simulink model "SimulacionControladorRechazoPerturbacion"  (R2023b)
settings: Solver=VariableStepAuto  StartTime=0.0  StopTime=30  RelTol=1e-3
values from neighbouring files (symbols this model uses):
  alfa_cu = 3.9E-3    (= 0.0039)    [Parametros.m]
  b_a = J_eq * n * omega_n    [MigracionPolosControladorExterno.m]    (also in Parametros.m = 1)
  b_eq = b_m + b_l/(r^2)    (= 2.19444444444e-05)    [Parametros.m]
  C_ts = 0.818    [Parametros.m]
  g = 9.80665    [Parametros.m]
  J_eq = J_m + J_l/(r^2)    [Parametros.m]
  k_l = m*l_cm + m_l(1)*l_l    [Parametros.m]
  K_sa = J_eq * n * omega_n^2    [MigracionPolosControladorExterno.m]    (also in Parametros.m = 1)
  K_sia = J_eq * omega_n^3    [MigracionPolosControladorExterno.m]    (also in Parametros.m = 1)
  Ke_int = 3.2768e10    (= 32768000000)    [Parametros.m]
  Ke_t = 6.4e3    (= 6400)    [Parametros.m]
  Ke_w = 1.024e7    (= 10240000)    [Parametros.m]
  L_d = 6.6E-3    (= 0.0066)    [Parametros.m]
  L_ls = 0.8E-3    (= 0.0008)    [Parametros.m]
  L_q = 5.8E-3    (= 0.0058)    [Parametros.m]
  lambda_m = 0.016    [Parametros.m]
  P_p = 3    [Parametros.m]
  r = 120    [MigracionPolosControladorExterno.m]    (also in Parametros.m)
  R_tsamb = 146.7    [Parametros.m]
  Rs_ref = 1.02    [Parametros.m]
  Tita_0 = 0    [Parametros.m]
  Ts_0 = 20    [Parametros.m]
  Tsref = 20    [Parametros.m]
settings Model: Creator=Home  LastModifiedBy=Home

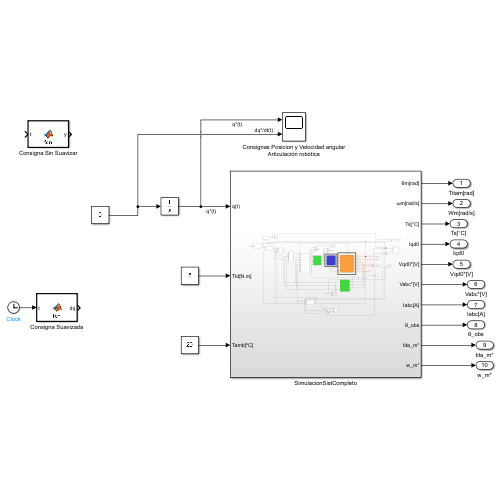
[thumbnail: Simulink's stored preview of the top-level diagram]
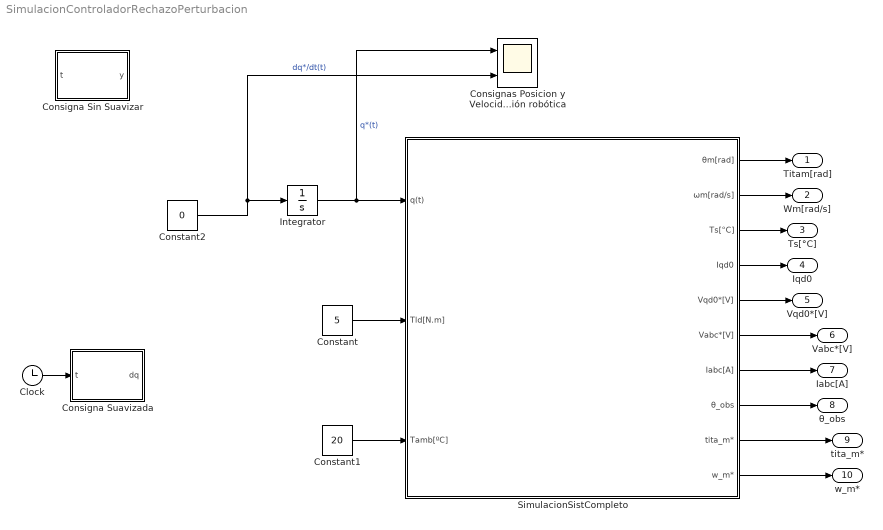
== system SimulacionControladorRechazoPerturbacion ==
  Clock : Clock
  Consigna Sin Suavizar : MATLAB Function  TreatAsAtomicUnit=on
  Consigna Suavizada : MATLAB Function  TreatAsAtomicUnit=on
  Consignas Posicion y Velocidad angular Articulación robótica : Scope  NumInputPorts=2
  Constant : Constant  Value=5
  Constant1 : Constant  Value=20
  Constant2 : Constant  Value=0
  Integrator : Integrator
  SimulacionSistCompleto : Subsystem
  Titam[rad] : Outport
  Wm[rad/s] : Outport  Port=2
  Ts[°C] : Outport  Port=3
  Iqd0 : Outport  Port=4
  Vqd0*[V] : Outport  Port=5
  Vabc*[V] : Outport  Port=6
  Iabc[A] : Outport  Port=7
  θ_obs : Outport  Port=8
  tita_m* : Outport  Port=9
  w_m* : Outport  Port=10
  wires:
  Constant2/1 -> Consignas Posicion y Velocidad angular Articulación robótica/2, Integrator/1  "dq*/dt(t)"
  Clock/1 -> Consigna Suavizada/1(t)
  SimulacionSistCompleto/4(Iqd0) -> Iqd0/1
  Constant/1 -> SimulacionSistCompleto/2(Tld[N.m])
  SimulacionSistCompleto/10(w_m*) -> w_m*/1
  SimulacionSistCompleto/9(tita_m*) -> tita_m*/1
  SimulacionSistCompleto/3(Ts[°C]) -> Ts[°C]/1
  SimulacionSistCompleto/2(ωm[rad/s]) -> Wm[rad/s]/1
  Constant1/1 -> SimulacionSistCompleto/3(Tamb[ºC])
  SimulacionSistCompleto/1(θm[rad]) -> Titam[rad]/1
  SimulacionSistCompleto/8(θ_obs) -> θ_obs/1
  SimulacionSistCompleto/5(Vqd0*[V]) -> Vqd0*[V]/1
  SimulacionSistCompleto/7(Iabc[A]) -> Iabc[A]/1
  SimulacionSistCompleto/6(Vabc*[V]) -> Vabc*[V]/1
  Integrator/1 -> Consignas Posicion y Velocidad angular Articulación robótica/1, SimulacionSistCompleto/1(q(t))  "q*(t)"

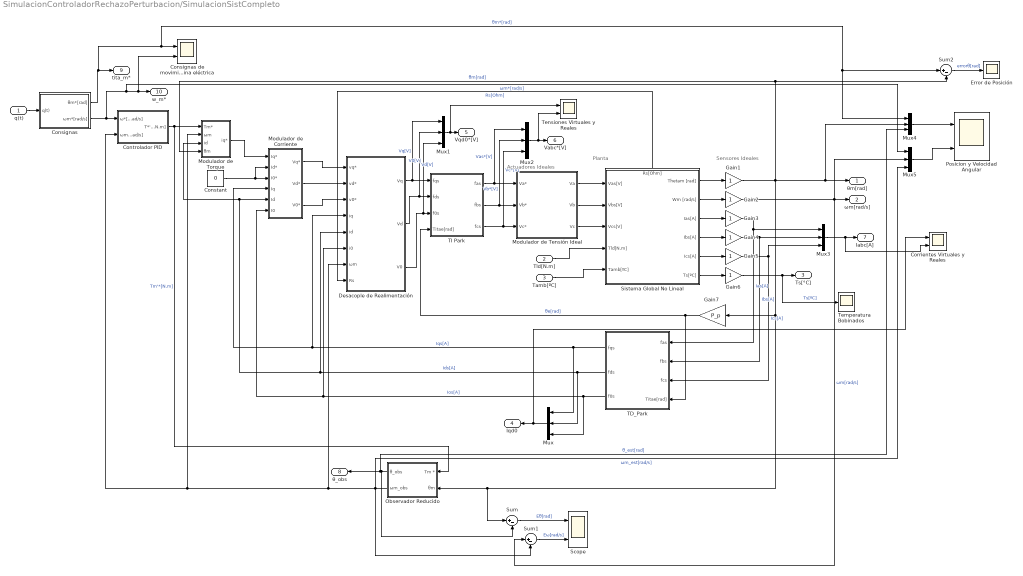
== system SimulacionControladorRechazoPerturbacion/SimulacionSistCompleto ==
  note: Actuadores Ideales
  note: Planta
  note: Sensores Ideales
  q(t) : Inport
  Tld[N.m] : Inport  Port=2
  Tamb[ºC] : Inport  Port=3
  Consignas : Subsystem
  Consignas de movimiento máquina eléctrica : Scope  NumInputPorts=2
  Constant : Constant  Value=0
  Controlador PID : Subsystem
  Corrientes Virtuales y Reales : Scope  NumInputPorts=2
  Desacople de Realimentación : Subsystem
  Error de Posición : Scope
  Gain{1..6} (6 alike) : Gain
  Gain7 : Gain  Gain=P_p
  Modulador de Corriente : Subsystem
  Modulador de Tensión Ideal : Subsystem
  Modulador de Torque : Subsystem
  Mux{,1..5} (6 alike) : Mux  Inputs=3
  Observador Reducido : Subsystem
  Posicion y Velocidad Angular : Scope  NumInputPorts=2
  Scope : Scope  NumInputPorts=2
  Sistema Global No Lineal : Subsystem
      settings: PortSchema="{\"entries\":[{\"content\":{\"sides\":[{\"content\":{\"connectorIds\":[\"In1\",\"In2\",\"In3\",\"In4\",\"In5\"]},\"type\":\"ConnectorPlacement.EquallySpacedRectSide\",\"uuid\":\"e69950d9-128a-479c-bb9c-058e9f1d4c4a\"},{\"content\":{\"connectorIds\":[\"Out1\",\"Out2\",\"Out3\",\"Out4\",\"Out5\",\"Out6\"],\"side\":\"RIGHT\"},\"type\":\"ConnectorPlacement.EquallySpacedRectSide\",\"uuid\":\"1754f544-d789-47dd-8fe5-32cce928f6e8\"},{\"content\":{\"connectorIds\":[\"Out7\"],\"side\":\"TOP\"},\"type\":\"ConnectorPlacement.EquallySpacedRectSide\",\"uuid\":\"429b420b-76ac-4d06-af5f-80d5ebf45ad3\"}]},\"type\":\"ConnectorPlacement.EquallySpacedConnector\",\"uuid\":\"839c6553-6053-4832-bfe9-eda0736393b8\"}],\"packageUris\":[\"http://schema.mathworks.com/mf0/Connector/R2020b\"],\"version\":\"1.0\"}"
  Sum : Sum  Inputs=|+-
  Sum1 : Sum  Inputs=|+-
  Sum2 : Sum  Inputs=|+-
  TD_Park : Subsystem
  TI Park : Subsystem
  Temperatura Bobinados : Scope
  Tensiones Virtuales y Reales : Scope  NumInputPorts=2
  θm[rad] : Outport
  ωm[rad/s] : Outport  Port=2
  Ts[°C] : Outport  Port=3
  Iqd0 : Outport  Port=4
  Vqd0*[V] : Outport  Port=5
  Vabc*[V] : Outport  Port=6
  Iabc[A] : Outport  Port=7
  θ_obs : Outport  Port=8
  tita_m* : Outport  Port=9
  w_m* : Outport  Port=10
  wires:
  Consignas/2(ωm*[rad/s]) -> Mux5/1, Consignas de movimiento máquina eléctrica/2, w_m*/1, Controlador PID/1(ω*[rad/s])  "ωm*[rad/s]"
  Modulador de Corriente/3(V0*) -> Desacople de Realimentación/3(v0*)
  Mux3/1 -> Corrientes Virtuales y Reales/2, Iabc[A]/1
  Sistema Global No Lineal/5(Ics[A]) -> Gain5/1
  Sistema Global No Lineal/1(Thetam [rad]) -> Gain1/1
  Gain1/1 -> Modulador de Torque/4(θm), Sum2/2, Mux4/2, θm[rad]/1, Gain7/1, Sum/1, Observador Reducido/2(θm)  "θm[rad]"
  TD_Park/2(fds) -> Modulador de Corriente/5(Id), Modulador de Torque/3(id), Desacople de Realimentación/5(id), Mux/2  "Ids[A]"
  TD_Park/1(fqs) -> Desacople de Realimentación/4(iq), Modulador de Corriente/4(Iq), Mux/1  "Iqs[A]"
  Gain5/1 -> Mux3/3, TD_Park/3(fcs)  "Ics[A]"
  Modulador de Tensión Ideal/3(Vc) -> Sistema Global No Lineal/3(Vcs[V])
  Modulador de Tensión Ideal/1(Va) -> Sistema Global No Lineal/1(Vas[V])
  Modulador de Torque/1(iq*) -> Modulador de Corriente/1(Iq*)
  Gain2/1 -> Mux5/2, Sum1/1, ωm[rad/s]/1  "ωm[rad/s]"
  Gain6/1 -> Ts[°C]/1, Temperatura Bobinados/1  "Ts[ºC]"
  TD_Park/3(f0s) -> Modulador de Corriente/6(I0), Desacople de Realimentación/6(i0), Mux/3  "Ios[A]"
  Modulador de Corriente/1(Vq*) -> Desacople de Realimentación/1(vq*)
  Desacople de Realimentación/2(Vd) -> Mux1/2, TI Park/2(fds)  "Vd[V]"
  Mux1/1 -> Tensiones Virtuales y Reales/1, Vqd0*[V]/1
  Gain3/1 -> TD_Park/1(fas), Mux3/1  "Ias[A]"
  Gain4/1 -> Mux3/2, TD_Park/2(fbs)  "Ibs[A]"
  Mux/1 -> Corrientes Virtuales y Reales/1, Iqd0/1
  TI Park/1(fas) -> Mux2/1, Modulador de Tensión Ideal/1(Va*)  "Vas*[V]"
  Gain7/1 -> TI Park/4(Titae[rad]), TD_Park/4(Titae[rad])  "θe[rad]"
  TI Park/3(fcs) -> Mux2/3, Modulador de Tensión Ideal/3(Vc*)  "Vc*[V]"
  Tld[N.m]/1 -> Sistema Global No Lineal/4(Tld[N.m])
  Mux2/1 -> Tensiones Virtuales y Reales/2, Vabc*[V]/1
  Sistema Global No Lineal/3(Ias[A]) -> Gain3/1
  Tamb[ºC]/1 -> Sistema Global No Lineal/5(Tamb[ºC])
  Desacople de Realimentación/1(Vq) -> Mux1/1, TI Park/1(fqs)  "Vq[V]"
  Modulador de Corriente/2(Vd*) -> Desacople de Realimentación/2(vd*)
  Desacople de Realimentación/3(V0) -> Mux1/3, TI Park/3(f0s)  "V0[V]"
  q(t)/1 -> Consignas/1(q(t))
  Sistema Global No Lineal/4(Ibs[A]) -> Gain4/1
  Constant/1 -> Modulador de Corriente/3(I0*), Modulador de Corriente/2(Id*)
  TI Park/2(fbs) -> Mux2/2, Modulador de Tensión Ideal/2("Vb* ")  "Vb*[V]"
  Modulador de Tensión Ideal/2(Vb) -> Sistema Global No Lineal/2(Vbs[V])
  Observador Reducido/1(θ_obs) -> Mux4/3, θ_obs/1, Sum/2  "θ_est[rad]"
  Sistema Global No Lineal/6(Ts[ºC]) -> Gain6/1
  Sistema Global No Lineal/2(Wm [rad/s]) -> Gain2/1
  Controlador PID/1(T*'m[N.m]) -> Modulador de Torque/1(Tm*), Observador Reducido/1(Tm *)  "Tm'*[N.m]"
  Observador Reducido/2(ωm_obs) -> Sum1/2, Mux5/3, Desacople de Realimentación/7(ωm), Modulador de Torque/2(ωm), Controlador PID/2(ωm[rad/s])  "ωm_est[rad/s]"
  Consignas/1(θm*[rad]) -> Sum2/1, Mux4/1, Consignas de movimiento máquina eléctrica/1, tita_m*/1  "θm*[rad]"
  Sistema Global No Lineal/7(Rs[Ohm]) -> Desacople de Realimentación/8(Rs)  "Rs[Ohm]"
  Mux4/1 -> Posicion y Velocidad Angular/1
  Mux5/1 -> Posicion y Velocidad Angular/2
  Sum/1 -> Scope/1  "Eθ[rad]"
  Sum1/1 -> Scope/2  "Eω[rad/s]"
  Sum2/1 -> Error de Posición/1  "errorθ[rad]"

== system SimulacionControladorRechazoPerturbacion/SimulacionSistCompleto/Consignas ==
  q(t) : Inport
  Derivative : Derivative
  Gain : Gain  Gain=r
  θm*[rad] : Outport
  ωm*[rad/s] : Outport  Port=2
  wires:
  Derivative/1 -> ωm*[rad/s]/1
  Gain/1 -> θm*[rad]/1, Derivative/1
  q(t)/1 -> Gain/1

== system SimulacionControladorRechazoPerturbacion/SimulacionSistCompleto/Controlador PID ==
  ω*[rad/s] : Inport
  ωm[rad/s] : Inport  Port=2
  Gain : Gain  Gain=b_a
  Gain1 : Gain  Gain=K_sia
  Gain2 : Gain  Gain=K_sa
  Integrator : Integrator
  Integrator1 : Integrator
  Sum : Sum  Inputs=|+-
  Sum1 : Sum  Inputs=+++
  T*'m[N.m] : Outport
  wires:
  Sum1/1 -> T*'m[N.m]/1
  Integrator1/1 -> Gain1/1
  ω*[rad/s]/1 -> Sum/1
  Sum/1 -> Gain/1, Integrator/1  "Ew"
  Gain2/1 -> Sum1/2
  Integrator/1 -> Integrator1/1, Gain2/1  "Eθ"
  ωm[rad/s]/1 -> Sum/2
  Gain/1 -> Sum1/3
  Gain1/1 -> Sum1/1

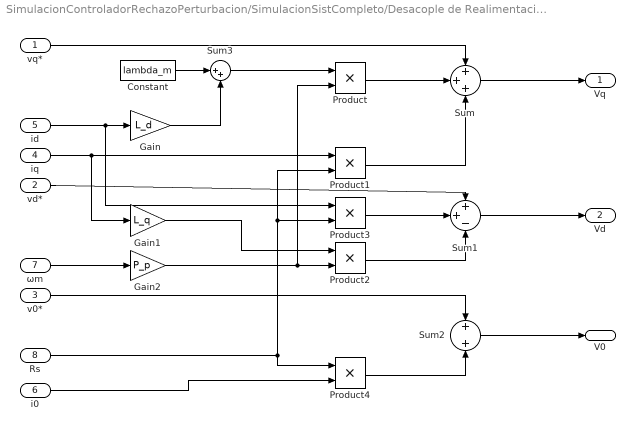
== system SimulacionControladorRechazoPerturbacion/SimulacionSistCompleto/Desacople de Realimentación ==
  vq* : Inport
  vd* : Inport  Port=2
  v0* : Inport  Port=3
  iq : Inport  Port=4
  id : Inport  Port=5
  i0 : Inport  Port=6
  ωm : Inport  Port=7
  Rs : Inport  Port=8
  Constant : Constant  Value=lambda_m
  Gain : Gain  Gain=L_d
  Gain1 : Gain  Gain=L_q
  Gain2 : Gain  Gain=P_p
  Product{,1..4} (5 alike) : Product
  Sum : Sum  Inputs=+++
  Sum1 : Sum  Inputs=++-
  Sum2 : Sum  Inputs=+|+
  Sum3 : Sum  Inputs=|++
  Vq : Outport
  Vd : Outport  Port=2
  V0 : Outport  Port=3
  wires:
  ωm/1 -> Gain2/1
  Sum/1 -> Vq/1
  Rs/1 -> Product4/1, Product1/2, Product3/2
  Gain/1 -> Sum3/2
  Product/1 -> Sum/2
  Sum2/1 -> V0/1
  Product4/1 -> Sum2/2
  Sum3/1 -> Product/1
  id/1 -> Product3/1, Gain/1
  vq*/1 -> Sum/1
  i0/1 -> Product4/2
  iq/1 -> Product1/1, Gain1/1
  Product2/1 -> Sum1/3
  Constant/1 -> Sum3/1
  v0*/1 -> Sum2/1
  Product1/1 -> Sum/3
  Gain2/1 -> Product/2, Product2/2
  vd*/1 -> Sum1/1
  Gain1/1 -> Product2/1
  Sum1/1 -> Vd/1
  Product3/1 -> Sum1/2

== system SimulacionControladorRechazoPerturbacion/SimulacionSistCompleto/Modulador de Corriente ==
  Iq* : Inport
  Id* : Inport  Port=2
  I0* : Inport  Port=3
  Iq : Inport  Port=4
  Id : Inport  Port=5
  I0 : Inport  Port=6
  Gain : Gain  Gain=5000*L_q
  Gain1 : Gain  Gain=5000*L_d
  Gain2 : Gain  Gain=5000*L_ls
  Sum : Sum  Inputs=|+-
  Sum1 : Sum  Inputs=|+-
  Sum2 : Sum  Inputs=|+-
  Vq* : Outport
  Vd* : Outport  Port=2
  V0* : Outport  Port=3
  wires:
  Gain2/1 -> V0*/1
  Sum/1 -> Gain/1
  Sum1/1 -> Gain1/1
  Gain/1 -> Vq*/1
  Iq/1 -> Sum/2
  I0*/1 -> Sum2/1
  Iq*/1 -> Sum/1
  Id/1 -> Sum1/2
  Sum2/1 -> Gain2/1
  Id*/1 -> Sum1/1
  Gain1/1 -> Vd*/1
  I0/1 -> Sum2/2

== system SimulacionControladorRechazoPerturbacion/SimulacionSistCompleto/Modulador de Tensión Ideal ==
  Va* : Inport
  "Vb* " : Inport  Port=2
  Vc* : Inport  Port=3
  Gain : Gain
  Gain1 : Gain
  Gain2 : Gain
  Va : Outport
  Vb : Outport  Port=2
  Vc : Outport  Port=3
  wires:
  Vc*/1 -> Gain2/1
  "Vb* "/1 -> Gain1/1
  Gain/1 -> Va/1
  Va*/1 -> Gain/1
  Gain1/1 -> Vb/1
  Gain2/1 -> Vc/1

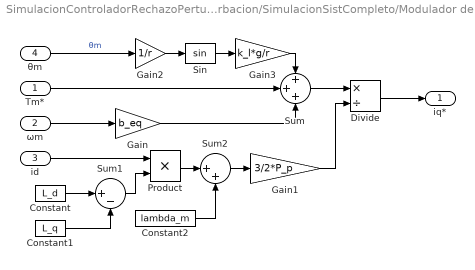
== system SimulacionControladorRechazoPerturbacion/SimulacionSistCompleto/Modulador de Torque ==
  Tm* : Inport
  ωm : Inport  Port=2
  id : Inport  Port=3
  θm : Inport  Port=4
  Constant : Constant  Value=L_d
  Constant1 : Constant  Value=L_q
  Constant2 : Constant  Value=lambda_m
  Divide : Product  Inputs=*/
  Gain : Gain  Gain=b_eq
  Gain1 : Gain  Gain=3/2*P_p
  Gain2 : Gain  Gain=1/r
  Gain3 : Gain  Gain=k_l*g/r
  Product : Product
  Sin : Trigonometry
  Sum : Sum  Inputs=+++
  Sum1 : Sum  Inputs=|+-
  Sum2 : Sum  Inputs=|++
  iq* : Outport
  wires:
  Constant2/1 -> Sum2/2
  ωm/1 -> Gain/1
  Sum1/1 -> Product/2
  Gain3/1 -> Sum/1
  θm/1 -> Gain2/1  "θm"
  Sum2/1 -> Gain1/1
  Constant/1 -> Sum1/1
  Gain1/1 -> Divide/2
  Divide/1 -> iq*/1
  Product/1 -> Sum2/1
  Gain/1 -> Sum/3
  Constant1/1 -> Sum1/2
  Sin/1 -> Gain3/1
  Gain2/1 -> Sin/1
  Sum/1 -> Divide/1
  id/1 -> Product/1
  Tm*/1 -> Sum/2

== system SimulacionControladorRechazoPerturbacion/SimulacionSistCompleto/Observador Reducido ==
  Tm * : Inport
  θm : Inport  Port=2
  Gain : Gain  Gain=1/J_eq
  Gain1 : Gain  Gain=Ke_int
  Gain10 : Gain  Gain=Ke_t
  Gain9 : Gain  Gain=Ke_w
  Integrator : Integrator
  Integrator1 : Integrator
  Integrator2 : Integrator
  Sum : Sum  Inputs=++|
  Sum1 : Sum  Inputs=++|
  Sum2 : Sum  Inputs=+|-
  Sum3 : Sum  Inputs=++|
  θ_obs : Outport
  ωm_obs : Outport  Port=2
  wires:
  Gain10/1 -> Sum1/1
  Sum2/1 -> Gain1/1, Gain9/1, Gain10/1
  Integrator1/1 -> θ_obs/1, Sum2/2
  Tm */1 -> Gain/1
  θm/1 -> Sum2/1
  Sum1/1 -> ωm_obs/1, Integrator1/1
  Integrator/1 -> Sum1/2
  Sum/1 -> Integrator/1
  Gain9/1 -> Sum/1
  Gain/1 -> Sum3/2
  Sum3/1 -> Sum/2
  Integrator2/1 -> Sum3/1
  Gain1/1 -> Integrator2/1

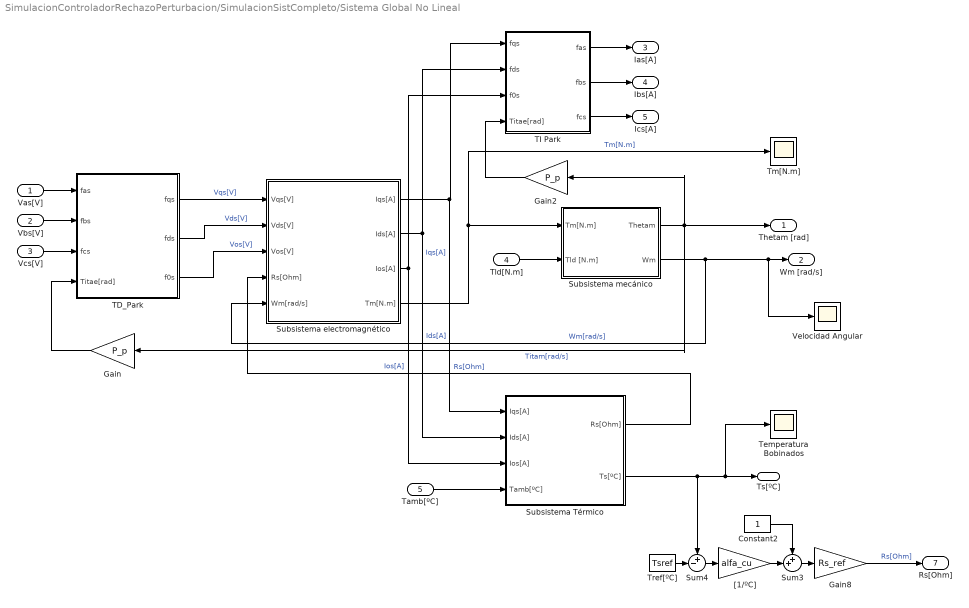
== system SimulacionControladorRechazoPerturbacion/SimulacionSistCompleto/Sistema Global No Lineal ==
  Vas[V] : Inport
  Vbs[V] : Inport  Port=2
  Vcs[V] : Inport  Port=3
  Tld[N.m] : Inport  Port=4
  Tamb[ºC] : Inport  Port=5
  Constant2 : Constant
  Gain : Gain  Gain=P_p
  Gain2 : Gain  Gain=P_p
  Gain8 : Gain  Gain=Rs_ref
  Subsistema Térmico : Subsystem
  Subsistema electromagnético : Subsystem
  Subsistema mecánico : Subsystem
  Sum3 : Sum  Inputs=++|
  Sum4 : Sum  Inputs=+-|
  TD_Park : Subsystem
  TI Park : Subsystem
  Temperatura Bobinados : Scope
  Tm[N.m] : Scope
  Tref[ºC] : Constant  Value=Tsref
  Velocidad Angular : Scope
  "[1/ºC]" : Gain  Gain=alfa_cu
  Thetam [rad] : Outport
  Wm [rad/s] : Outport  Port=2
  Ias[A] : Outport  Port=3
  Ibs[A] : Outport  Port=4
  Ics[A] : Outport  Port=5
  Ts[ºC] : Outport  Port=6
  Rs[Ohm] : Outport  Port=7
  wires:
  Subsistema electromagnético/3(Ios[A]) -> Subsistema Térmico/3(Ios[A]), TI Park/3(f0s)  "Ios[A]"
  Subsistema mecánico/2(Wm) -> Velocidad Angular/1, Wm [rad/s]/1, Subsistema electromagnético/5(Wm[rad/s])  "Wm[rad/s]"
  TD_Park/3(f0s) -> Subsistema electromagnético/3(Vos[V])  "Vos[V]"
  Gain/1 -> TD_Park/4(Titae[rad])
  Subsistema Térmico/1(Rs[Ohm]) -> Subsistema electromagnético/4(Rs[Ohm])  "Rs[Ohm]"
  TD_Park/1(fqs) -> Subsistema electromagnético/1(Vqs[V])  "Vqs[V]"
  Vbs[V]/1 -> TD_Park/2(fbs)
  Vcs[V]/1 -> TD_Park/3(fcs)
  Subsistema electromagnético/1(Iqs[A]) -> Subsistema Térmico/1(Iqs[A]), TI Park/1(fqs)  "Iqs[A]"
  Subsistema electromagnético/4(Tm[N.m]) -> Tm[N.m]/1, Subsistema mecánico/1(Tm[N.m])  "Tm[N.m]"
  Subsistema mecánico/1(Thetam) -> Thetam [rad]/1, Gain2/1, Gain/1  "Titam[rad/s]"
  Tamb[ºC]/1 -> Subsistema Térmico/4(Tamb[ºC])
  Vas[V]/1 -> TD_Park/1(fas)
  TD_Park/2(fds) -> Subsistema electromagnético/2(Vds[V])  "Vds[V]"
  TI Park/2(fbs) -> Ibs[A]/1
  Subsistema electromagnético/2(Ids[A]) -> TI Park/2(fds), Subsistema Térmico/2(Ids[A])  "Ids[A]"
  Gain2/1 -> TI Park/4(Titae[rad])
  TI Park/1(fas) -> Ias[A]/1
  Subsistema Térmico/2(Ts[ºC]) -> Sum4/1, Temperatura Bobinados/1, Ts[ºC]/1
  Tld[N.m]/1 -> Subsistema mecánico/2(Tld [N.m])
  TI Park/3(fcs) -> Ics[A]/1
  "[1/ºC]"/1 -> Sum3/2
  Sum3/1 -> Gain8/1
  Tref[ºC]/1 -> Sum4/2
  Constant2/1 -> Sum3/1
  Sum4/1 -> "[1/ºC]"/1
  Gain8/1 -> Rs[Ohm]/1  "Rs[Ohm]"

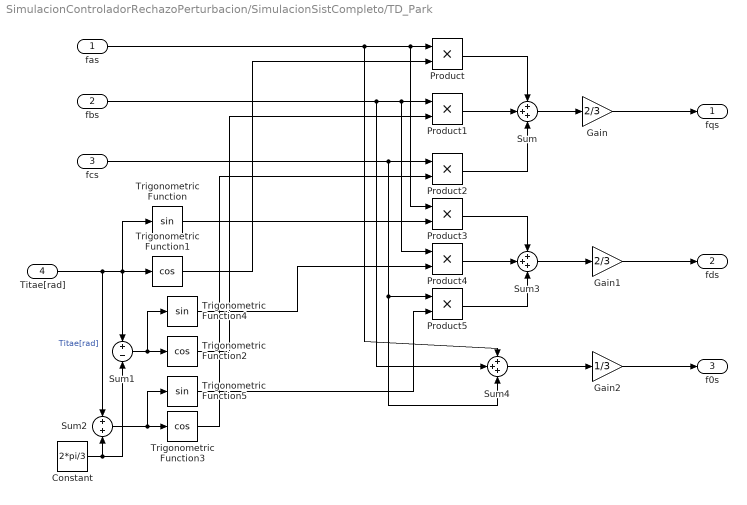
== system SimulacionControladorRechazoPerturbacion/SimulacionSistCompleto/TD_Park ==
  fas : Inport
  fbs : Inport  Port=2
  fcs : Inport  Port=3
  Titae[rad] : Inport  Port=4
  Constant : Constant  Value=2*pi/3
  Gain : Gain  Gain=2/3
  Gain1 : Gain  Gain=2/3
  Gain2 : Gain  Gain=1/3
  Product{,1..5} (6 alike) : Product
  Sum : Sum  Inputs=+++
  Sum1 : Sum  Inputs=+-
  Sum2 : Sum
  Sum3 : Sum  Inputs=+++
  Sum4 : Sum  Inputs=+++
  Trigonometric Function : Trigonometry
  Trigonometric Function1 : Trigonometry  Operator=cos
  Trigonometric Function2 : Trigonometry  Operator=cos
  Trigonometric Function3 : Trigonometry  Operator=cos
  Trigonometric Function4 : Trigonometry
  Trigonometric Function5 : Trigonometry
  fqs : Outport
  fds : Outport  Port=2
  f0s : Outport  Port=3
  wires:
  fas/1 -> Sum4/1, Product3/1, Product/1
  Trigonometric Function3/1 -> Product2/2
  Sum1/1 -> Trigonometric Function4/1, Trigonometric Function2/1
  Constant/1 -> Sum2/2, Sum1/2
  Trigonometric Function1/1 -> Product/2
  fcs/1 -> Product5/1, Sum4/3, Product2/1
  Product5/1 -> Sum3/3
  Product/1 -> Sum/1
  Product3/1 -> Sum3/1
  Product1/1 -> Sum/2
  Trigonometric Function/1 -> Product3/2
  Sum2/1 -> Trigonometric Function5/1, Trigonometric Function3/1
  Trigonometric Function5/1 -> Product5/2
  Sum4/1 -> Gain2/1
  fbs/1 -> Sum4/2, Product4/1, Product1/1
  Product2/1 -> Sum/3
  Gain/1 -> fqs/1
  Trigonometric Function4/1 -> Product4/2
  Product4/1 -> Sum3/2
  Trigonometric Function2/1 -> Product1/2
  Gain2/1 -> f0s/1
  Sum/1 -> Gain/1
  Gain1/1 -> fds/1
  Sum3/1 -> Gain1/1
  Titae[rad]/1 -> Sum2/1, Trigonometric Function/1, Sum1/1, Trigonometric Function1/1  "Titae[rad]"

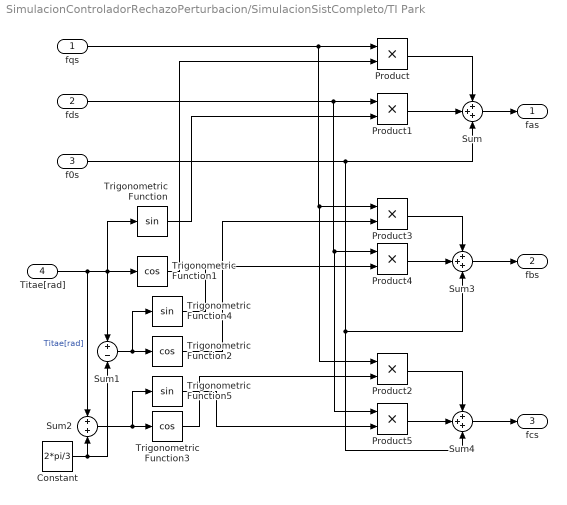
== system SimulacionControladorRechazoPerturbacion/SimulacionSistCompleto/TI Park ==
  fqs : Inport
  fds : Inport  Port=2
  f0s : Inport  Port=3
  Titae[rad] : Inport  Port=4
  Constant : Constant  Value=2*pi/3
  Product{,1..5} (6 alike) : Product
  Sum : Sum  Inputs=+++
  Sum1 : Sum  Inputs=+-
  Sum2 : Sum
  Sum3 : Sum  Inputs=+++
  Sum4 : Sum  Inputs=+++
  Trigonometric Function : Trigonometry
  Trigonometric Function1 : Trigonometry  Operator=cos
  Trigonometric Function2 : Trigonometry  Operator=cos
  Trigonometric Function3 : Trigonometry  Operator=cos
  Trigonometric Function4 : Trigonometry
  Trigonometric Function5 : Trigonometry
  fas : Outport
  fbs : Outport  Port=2
  fcs : Outport  Port=3
  wires:
  Constant/1 -> Sum2/2, Sum1/2
  Product1/1 -> Sum/2
  Trigonometric Function2/1 -> Product3/2
  Trigonometric Function5/1 -> Product5/2
  fds/1 -> Product1/1, Product5/1, Product4/1
  f0s/1 -> Sum/3, Sum3/3, Sum4/3
  Product3/1 -> Sum3/1
  fqs/1 -> Product/1, Product2/1, Product3/1
  Product2/1 -> Sum4/1
  Trigonometric Function1/1 -> Product/2
  Product/1 -> Sum/1
  Sum2/1 -> Trigonometric Function5/1, Trigonometric Function3/1
  Sum1/1 -> Trigonometric Function4/1, Trigonometric Function2/1
  Trigonometric Function/1 -> Product1/2
  Product4/1 -> Sum3/2
  Sum/1 -> fas/1
  Trigonometric Function3/1 -> Product2/2
  Product5/1 -> Sum4/2
  Trigonometric Function4/1 -> Product4/2
  Sum3/1 -> fbs/1
  Sum4/1 -> fcs/1
  Titae[rad]/1 -> Sum2/1, Trigonometric Function/1, Sum1/1, Trigonometric Function1/1  "Titae[rad]"

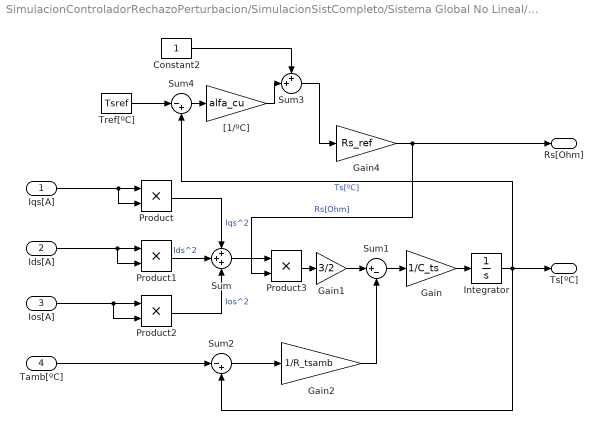
== system SimulacionControladorRechazoPerturbacion/SimulacionSistCompleto/Sistema Global No Lineal/Subsistema Térmico ==
  Iqs[A] : Inport
  Ids[A] : Inport  Port=2
  Ios[A] : Inport  Port=3
  Tamb[ºC] : Inport  Port=4
  Constant2 : Constant
  Gain : Gain  Gain=1/C_ts
  Gain1 : Gain  Gain=3/2
  Gain2 : Gain  Gain=1/R_tsamb
  Gain4 : Gain  Gain=Rs_ref
  Integrator : Integrator  InitialCondition=Ts_0
  Product{,1..3} (4 alike) : Product
  Sum : Sum  Inputs=+++
  Sum1 : Sum  Inputs=|+-
  Sum2 : Sum  Inputs=|-+
  Sum3 : Sum  Inputs=++|
  Sum4 : Sum  Inputs=|-+
  Tref[ºC] : Constant  Value=Tsref
  "[1/ºC]" : Gain  Gain=alfa_cu
  Rs[Ohm] : Outport
  Ts[ºC] : Outport  Port=2
  wires:
  Sum3/1 -> Gain4/1
  Gain/1 -> Integrator/1
  Product1/1 -> Sum/2  "Ids^2"
  Product/1 -> Sum/1  "Iqs^2"
  Sum/1 -> Product3/1
  Iqs[A]/1 -> Product/2, Product/1
  Ids[A]/1 -> Product1/2, Product1/1
  Product2/1 -> Sum/3  "Ios^2"
  Sum4/1 -> "[1/ºC]"/1
  Tamb[ºC]/1 -> Sum2/1
  Sum1/1 -> Gain/1
  Sum2/1 -> Gain2/1
  Gain4/1 -> Rs[Ohm]/1, Product3/2  "Rs[Ohm]"
  Gain1/1 -> Sum1/1
  Ios[A]/1 -> Product2/2, Product2/1
  Constant2/1 -> Sum3/1
  Tref[ºC]/1 -> Sum4/1
  Product3/1 -> Gain1/1
  "[1/ºC]"/1 -> Sum3/2
  Gain2/1 -> Sum1/2
  Integrator/1 -> Ts[ºC]/1, Sum2/2, Sum4/2  "Ts[ºC]"

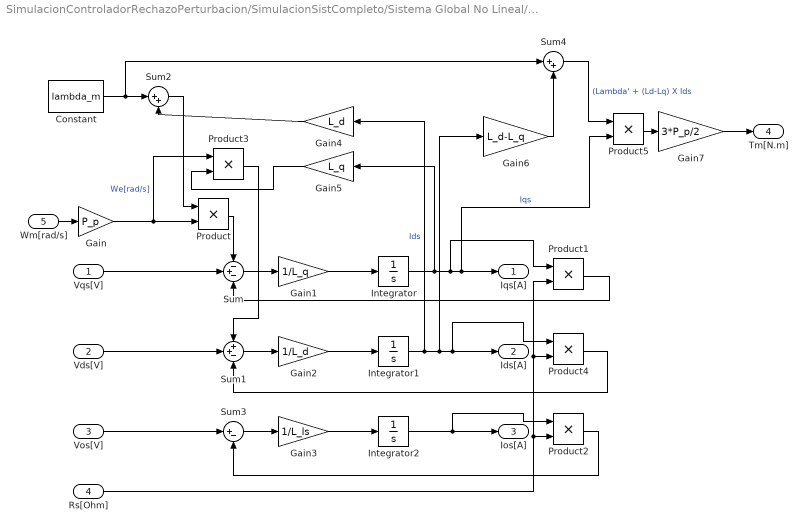
== system SimulacionControladorRechazoPerturbacion/SimulacionSistCompleto/Sistema Global No Lineal/Subsistema electromagnético ==
  Vqs[V] : Inport
  Vds[V] : Inport  Port=2
  Vos[V] : Inport  Port=3
  Rs[Ohm] : Inport  Port=4
  Wm[rad/s] : Inport  Port=5
  Constant : Constant  Value=lambda_m
  Gain : Gain  Gain=P_p
  Gain1 : Gain  Gain=1/L_q
  Gain2 : Gain  Gain=1/L_d
  Gain3 : Gain  Gain=1/L_ls
  Gain4 : Gain  Gain=L_d
  Gain5 : Gain  Gain=L_q
  Gain6 : Gain  Gain=L_d-L_q
  Gain7 : Gain  Gain=3*P_p/2
  Integrator : Integrator
  Integrator1 : Integrator  InitialCondition=-0.5
  Integrator2 : Integrator
  Product{,1..5} (6 alike) : Product
  Sum : Sum  Inputs=-+-
  Sum1 : Sum  Inputs=++-
  Sum2 : Sum  Inputs=|++
  Sum3 : Sum  Inputs=|+-
  Sum4 : Sum  Inputs=|++
  Iqs[A] : Outport
  Ids[A] : Outport  Port=2
  Ios[A] : Outport  Port=3
  Tm[N.m] : Outport  Port=4
  wires:
  Product3/1 -> Sum1/1
  Gain5/1 -> Product3/2
  Vos[V]/1 -> Sum3/1
  Sum1/1 -> Gain2/1
  Integrator/1 -> Gain5/1, Product1/1, Iqs[A]/1, Product5/2  "Iqs"
  Integrator2/1 -> Ios[A]/1, Product2/1
  Rs[Ohm]/1 -> Product4/2, Product1/2, Product2/2
  Product1/1 -> Sum/3
  Sum/1 -> Gain1/1
  Sum4/1 -> Product5/1  "(Lambda' + (Ld-Lq) X Ids"
  Integrator1/1 -> Gain6/1, Ids[A]/1, Product4/1, Gain4/1  "Ids"
  Gain/1 -> Product/2, Product3/1  "We[rad/s]"
  Sum3/1 -> Gain3/1
  Gain6/1 -> Sum4/2
  Wm[rad/s]/1 -> Gain/1
  Gain7/1 -> Tm[N.m]/1
  Product5/1 -> Gain7/1
  Vqs[V]/1 -> Sum/2
  Gain2/1 -> Integrator1/1
  Product/1 -> Sum/1
  Constant/1 -> Sum4/1, Sum2/1
  Sum2/1 -> Product/1
  Vds[V]/1 -> Sum1/2
  Gain4/1 -> Sum2/2
  Product4/1 -> Sum1/3
  Product2/1 -> Sum3/2
  Gain1/1 -> Integrator/1
  Gain3/1 -> Integrator2/1

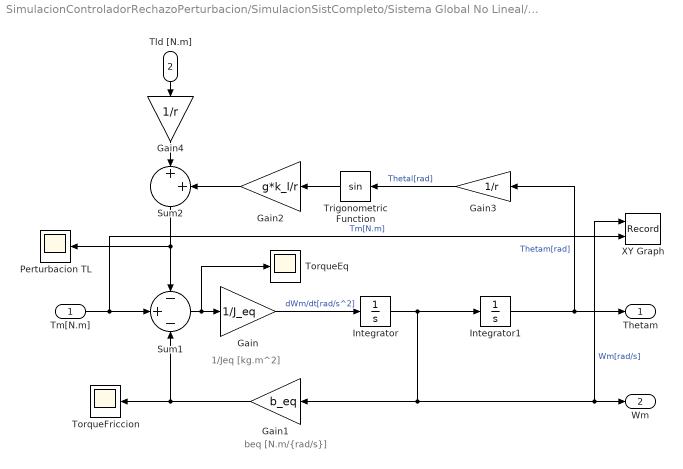
== system SimulacionControladorRechazoPerturbacion/SimulacionSistCompleto/Sistema Global No Lineal/Subsistema mecánico ==
  note: beq [N.m/{rad/s}]
  note: 1/Jeq [kg.m^2]
  Tm[N.m] : Inport
  Tld [N.m] : Inport  Port=2
  Gain : Gain  Gain=1/J_eq
  Gain1 : Gain  Gain=b_eq
  Gain2 : Gain  Gain=g*k_l/r
  Gain3 : Gain  Gain=1/r
  Gain4 : Gain  Gain=1/r
  Integrator : Integrator
  Integrator1 : Integrator  InitialCondition=Tita_0
  Perturbacion TL : Scope
  Sum1 : Sum  Inputs=-+-
  Sum2 : Sum  Inputs=|++
  TorqueEq : Scope
  TorqueFriccion : Scope
  Trigonometric Function : Trigonometry
  XY Graph : Record  FileSettingsInternal="{\"entries\":[{\"content\":{\"excelSettings\":{\"content\":{},\"type\":\"Streamout.ExcelSettings\"}},\"type\":\"Streamout.FileSettingStorage\",\"uuid\":\"\"}],\"packageUris\":[\"http:\\/\\/schema.mathworks.com\\/mf0\\/streamout_blocks\\/R2020a\"],\"version\":\"1.0\"}"  Layout=[1 1]  SignalsInternal="{\"entries\":[{\"content\":{\"signals\":[{\"content\":{\"blockPath\":[],\"dimensions\":[1],\"domain\":\"\",\"lineColor\":\"#a2142f\",\"port\":1,\"sid\":[\"\"],\"signalID\":93456,\"signalName\":\"Wm[rad\\/s]\"},\"type\":\"RecordBlkView.Signal\",\"uuid\":\"\"},{\"content\":{\"blockPath\":[],\"dimensions\":[1],\"domain\":\"\",\"lineColor\":\"#139fff\",\"port\":2,\"sid\":[\"\"],\"signalID\":93460,\"signalName\":\"Tm[N.m]\"},\"type\":\"RecordBlkView.Signal\",\"uuid\":\"\"}]},\"type\":\"RecordBlkView.InputSignals\",\"uuid\":\"\"}],\"packageUris\":[\"http:\\/\\/schema.mathworks.com\\/mf0\\/streamout_blocks\\/R2020a\"],\"version\":\"1.0\"}"  VisualizationBindings="{\"xyplotplugin\":{\"info\":[{\"series\":[],\"subplotID\":1}]}}"  CompatibilityTag=XY
  Thetam : Outport
  Wm : Outport  Port=2
  wires:
  Tld [N.m]/1 -> Gain4/1
  Gain3/1 -> Trigonometric Function/1  "Thetal[rad]"
  Tm[N.m]/1 -> XY Graph/2, Sum1/2  "Tm[N.m]"
  Integrator/1 -> XY Graph/1, Wm/1, Gain1/1, Integrator1/1  "Wm[rad/s]"
  Integrator1/1 -> Thetam/1, Gain3/1  "Thetam[rad]"
  Trigonometric Function/1 -> Gain2/1
  Gain1/1 -> TorqueFriccion/1, Sum1/3
  Gain/1 -> Integrator/1  "dWm/dt[rad/s^2]"
  Sum1/1 -> TorqueEq/1, Gain/1
  Gain4/1 -> Sum2/1
  Gain2/1 -> Sum2/2
  Sum2/1 -> Perturbacion TL/1, Sum1/1

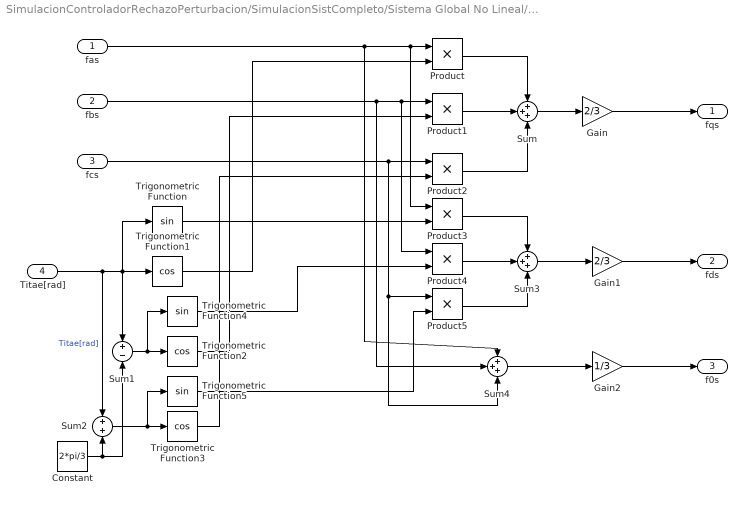
== system SimulacionControladorRechazoPerturbacion/SimulacionSistCompleto/Sistema Global No Lineal/TD_Park ==
  fas : Inport
  fbs : Inport  Port=2
  fcs : Inport  Port=3
  Titae[rad] : Inport  Port=4
  Constant : Constant  Value=2*pi/3
  Gain : Gain  Gain=2/3
  Gain1 : Gain  Gain=2/3
  Gain2 : Gain  Gain=1/3
  Product{,1..5} (6 alike) : Product
  Sum : Sum  Inputs=+++
  Sum1 : Sum  Inputs=+-
  Sum2 : Sum
  Sum3 : Sum  Inputs=+++
  Sum4 : Sum  Inputs=+++
  Trigonometric Function : Trigonometry
  Trigonometric Function1 : Trigonometry  Operator=cos
  Trigonometric Function2 : Trigonometry  Operator=cos
  Trigonometric Function3 : Trigonometry  Operator=cos
  Trigonometric Function4 : Trigonometry
  Trigonometric Function5 : Trigonometry
  fqs : Outport
  fds : Outport  Port=2
  f0s : Outport  Port=3
  wires:
  fas/1 -> Sum4/1, Product3/1, Product/1
  Trigonometric Function3/1 -> Product2/2
  Sum1/1 -> Trigonometric Function4/1, Trigonometric Function2/1
  Constant/1 -> Sum2/2, Sum1/2
  Trigonometric Function1/1 -> Product/2
  fcs/1 -> Product5/1, Sum4/3, Product2/1
  Product5/1 -> Sum3/3
  Product/1 -> Sum/1
  Product3/1 -> Sum3/1
  Product1/1 -> Sum/2
  Trigonometric Function/1 -> Product3/2
  Sum2/1 -> Trigonometric Function5/1, Trigonometric Function3/1
  Trigonometric Function5/1 -> Product5/2
  Sum4/1 -> Gain2/1
  fbs/1 -> Sum4/2, Product4/1, Product1/1
  Product2/1 -> Sum/3
  Gain/1 -> fqs/1
  Trigonometric Function4/1 -> Product4/2
  Product4/1 -> Sum3/2
  Trigonometric Function2/1 -> Product1/2
  Gain2/1 -> f0s/1
  Sum/1 -> Gain/1
  Gain1/1 -> fds/1
  Sum3/1 -> Gain1/1
  Titae[rad]/1 -> Sum2/1, Trigonometric Function/1, Sum1/1, Trigonometric Function1/1  "Titae[rad]"

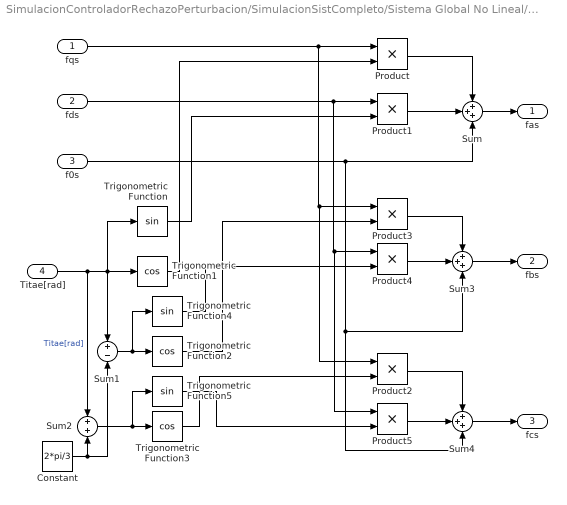
== system SimulacionControladorRechazoPerturbacion/SimulacionSistCompleto/Sistema Global No Lineal/TI Park ==
  fqs : Inport
  fds : Inport  Port=2
  f0s : Inport  Port=3
  Titae[rad] : Inport  Port=4
  Constant : Constant  Value=2*pi/3
  Product{,1..5} (6 alike) : Product
  Sum : Sum  Inputs=+++
  Sum1 : Sum  Inputs=+-
  Sum2 : Sum
  Sum3 : Sum  Inputs=+++
  Sum4 : Sum  Inputs=+++
  Trigonometric Function : Trigonometry
  Trigonometric Function1 : Trigonometry  Operator=cos
  Trigonometric Function2 : Trigonometry  Operator=cos
  Trigonometric Function3 : Trigonometry  Operator=cos
  Trigonometric Function4 : Trigonometry
  Trigonometric Function5 : Trigonometry
  fas : Outport
  fbs : Outport  Port=2
  fcs : Outport  Port=3
  wires:
  Constant/1 -> Sum2/2, Sum1/2
  Product1/1 -> Sum/2
  Trigonometric Function2/1 -> Product3/2
  Trigonometric Function5/1 -> Product5/2
  fds/1 -> Product1/1, Product5/1, Product4/1
  f0s/1 -> Sum/3, Sum3/3, Sum4/3
  Product3/1 -> Sum3/1
  fqs/1 -> Product/1, Product2/1, Product3/1
  Product2/1 -> Sum4/1
  Trigonometric Function1/1 -> Product/2
  Product/1 -> Sum/1
  Sum2/1 -> Trigonometric Function5/1, Trigonometric Function3/1
  Sum1/1 -> Trigonometric Function4/1, Trigonometric Function2/1
  Trigonometric Function/1 -> Product1/2
  Product4/1 -> Sum3/2
  Sum/1 -> fas/1
  Trigonometric Function3/1 -> Product2/2
  Product5/1 -> Sum4/2
  Trigonometric Function4/1 -> Product4/2
  Sum3/1 -> fbs/1
  Sum4/1 -> fcs/1
  Titae[rad]/1 -> Sum2/1, Trigonometric Function/1, Sum1/1, Trigonometric Function1/1  "Titae[rad]"

== matlab function SimulacionControladorRechazoPerturbacion/Consigna Suavizada ==
  data: t input; dq output
function dq  = fcn(t)
    % Salidas:
    % q  -> Consigna de posición [rad]
    % dq -> Consigna de velocidad [rad/s]
    
    % Constantes
    max_pos = 2 * pi;       % Posición máxima [rad]
    ramp_time = 0.1;       % Tiempo de rampa [s]
    plateau_time = 5;       % Duración de velocidad constante [s]
    total_time = 2 * plateau_time + 2 * ramp_time; % Tiempo total [s]
    
    % Velocidad máxima
    max_vel = max_pos / plateau_time; % Velocidad constante [rad/s]
    
    % Inicialización de variables de salida
    dq = 0; % Velocidad
    q = 0;  % Posición
    
    % Lógica de perfil de velocidad
    if t < ramp_time
        % Rampa de aceleración (inicio de movimiento)
        dq = max_vel * (t / ramp_time);
    elseif t >= ramp_time && t < plateau_time + ramp_time
        % Velocidad constante positiva (incremento lineal de posición)
        dq = max_vel;
    elseif t >= plateau_time + ramp_time && t < plateau_time + 2 * ramp_time
        % Rampa de desaceleración positiva (fin del incremento)
        dq = max_vel * (1 - (t - plateau_time - ramp_time) / ramp_time);
    elseif t >= plateau_time + 2 * ramp_time && t < 2 * plateau_time + 2 * ramp_time
        % Velocidad cero (mantener posición constante en 2*pi)
        dq = 0;
    elseif t >= 2 * plateau_time + 2 * ramp_time && t < 2 * plateau_time + 3 * ramp_time
        % Rampa de aceleración negativa (inicio del decremento)
        dq = -max_vel * ((t - 2 * plateau_time - 2 * ramp_time) / ramp_time);
    elseif t >= 2 * plateau_time + 3 * ramp_time && t < 3 * plateau_time + 3 * ramp_time
        % Velocidad constante negativa (decremento lineal de posición)
        dq = -max_vel;
    elseif t >= 3 * plateau_time + 3 * ramp_time && t < 3 * plateau_time + 4 * ramp_time
        % Rampa de desaceleración negativa (fin del decremento)
        dq = -max_vel * (1 - (t - 3 * plateau_time - 3 * ramp_time) / ramp_time);
    else
        % Fuera del rango definido, posición constante en 0
        dq = 0;
    end

end

== matlab function SimulacionControladorRechazoPerturbacion/Consigna Sin Suavizar ==
  data: t input; y output
function y = fcn(t)
    % Constantes
    max_pos = 2 * pi;       % Posición máxima (2*pi)
    ramp_time = 5;          % Tiempo de rampa ascendente y descendente
    stable_time = 10;       % Tiempo en que la posición se mantiene estable

    if t >= 0 && t < ramp_time
        % Rampa ascendente
        y = (max_pos / ramp_time) * t;
    elseif t >= ramp_time && t < stable_time
        % Posición estable
        y = max_pos;
    elseif t >= stable_time && t < stable_time + ramp_time
        % Rampa descendente
        y = max_pos - (max_pos / ramp_time) * (t - stable_time);
    else
        % Fuera del rango definido
        y = 0;
    end
end
